simulink model "Stateflow_SD24b"  (R2015b)
settings: Solver=VariableStepAuto  StartTime=0.0  StopTime=inf  RelTol=1e-3
settings Model: Creator=amyyang  LastModifiedBy=amyyang

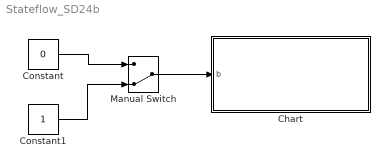
== system Stateflow_SD24b ==
  Chart : Stateflow chart  TreatAsAtomicUnit=on
  Constant : Constant  Value=0
  Constant1 : Constant
  Manual Switch : ManualSwitch  CurrentSetting=0
  wires:
  Manual Switch/1 -> Chart/1(b)
  Constant1/1 -> Manual Switch/2
  Constant/1 -> Manual Switch/1

== stateflow chart Stateflow_SD24b/Chart ==
  state B
    state BB1
    state BB2
    (default) -> BB1 [order 1]
    BB1 -> BB2 : after(5,sec)
    BB2 -> BB1 : after(5,sec)
    (default) -> BB2 [order 2]
  state A
  (default) -> A
  A -> B : [ b > 0]
  data: b input
